simulink model "block_diagram"  (R2016b)
settings: Solver=VariableStepAuto  StartTime=0.0  StopTime=10.0  RelTol=1e-3
libraries: simulink x6
settings Model: Creator=sorinalupu  LastModifiedBy=sorinalupu

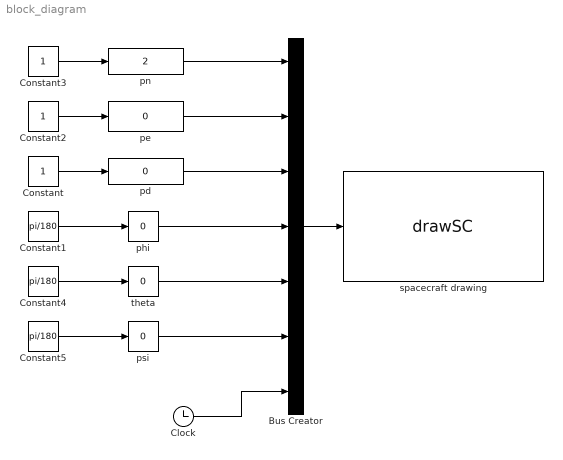
== system block_diagram ==
  Bus Creator : BusCreator  Inputs=7
  Clock : Clock
  Constant : Constant
  Constant1 : Constant  Value=pi/180
  Constant2 : Constant
  Constant3 : Constant
  Constant4 : Constant  Value=pi/180
  Constant5 : Constant  Value=pi/180
  pd : simulink/Math Operations/Slider Gain  low=-3  gain=0  high=3
  pe : simulink/Math Operations/Slider Gain  low=-3  gain=0  high=3
  "phi " : simulink/Math Operations/Slider Gain  low=0  gain=0  high=180
  "pn " : simulink/Math Operations/Slider Gain  low=-3  gain=2  high=3
  psi : simulink/Math Operations/Slider Gain  low=0  gain=0  high=180
  spacecraft drawing : MATLABFcn  MATLABFcn=drawSC  OutputDimensions=0  OutputSignalType=real
  theta : simulink/Math Operations/Slider Gain  low=0  gain=0  high=180
  wires:
  Bus Creator/1 -> spacecraft drawing/1
  Constant/1 -> pd/1
  Constant1/1 -> "phi "/1
  Clock/1 -> Bus Creator/7
  Constant3/1 -> "pn "/1
  Constant2/1 -> pe/1
  "phi "/1 -> Bus Creator/4
  "pn "/1 -> Bus Creator/1
  pe/1 -> Bus Creator/2
  pd/1 -> Bus Creator/3
  Constant4/1 -> theta/1
  Constant5/1 -> psi/1
  theta/1 -> Bus Creator/5
  psi/1 -> Bus Creator/6
